simulink model "untitled2"  (R2020b)
settings: Solver=VariableStepAuto  StartTime=0.0  StopTime=10.0  RelTol=1e-3
libraries: neural x2
settings Model: Creator=Danik  LastModifiedBy=Danik

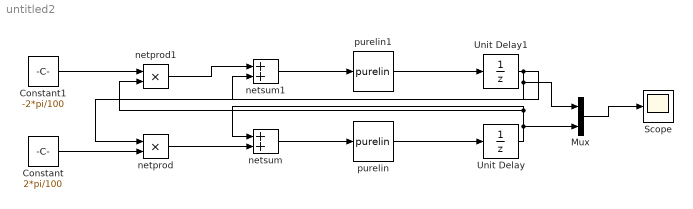
== system untitled2 ==
  Constant : Constant  Value=2*pi/100
  Constant1 : Constant  Value=-2*pi/100
  Mux : Mux  Inputs=2
  Scope : Scope
  Unit Delay : UnitDelay  InitialCondition=-1  SampleTime=2*pi/100  HasFrameUpgradeWarning=on
  Unit Delay1 : UnitDelay  InitialCondition=-1  SampleTime=2*pi/100  HasFrameUpgradeWarning=on
  netprod : Product  InputSameDT=on  RndMeth=Zero  SaturateOnIntegerOverflow=on  OutDataTypeStr=Inherit: Same as first input
  netprod1 : Product  InputSameDT=on  RndMeth=Zero  SaturateOnIntegerOverflow=on  OutDataTypeStr=Inherit: Same as first input
  netsum : Sum  Inputs=2  InputSameDT=on  SaturateOnIntegerOverflow=on  OutDataTypeStr=Inherit: Same as first input
  netsum1 : Sum  Inputs=2  InputSameDT=on  SaturateOnIntegerOverflow=on  OutDataTypeStr=Inherit: Same as first input
  purelin : neural/Transfer Functions/purelin
  purelin1 : neural/Transfer Functions/purelin
  wires:
  Constant/1 -> netprod/2
  Constant1/1 -> netprod1/1
  netprod1/1 -> netsum1/1
  netprod/1 -> netsum/2
  netsum/1 -> purelin/1
  netsum1/1 -> purelin1/1
  purelin/1 -> Unit Delay/1
  purelin1/1 -> Unit Delay1/1
  Unit Delay/1 -> Mux/2, netprod1/2, netsum/1
  Unit Delay1/1 -> Mux/1, netprod/1, netsum1/2
  Mux/1 -> Scope/1
